simulink model "Optimization_Implementation_Sept1_2021"  (R2021a)
settings: Solver=FixedStepAuto  StartTime=0.0  StopTime=inf  FixedStep=.001  RelTol=1e-3
libraries: speedgoatlib_IO691 x5, canmsglib x4, slrealtimeutilitieslib x2
settings Model: SimulationMode=external  NumberOfSteps=2  Creator=celwe  LastModifiedBy=celwe
settings SolverCC: ConcurrentTasks=on  PositivePriorityOrder=on
settings OptimizationCC: BlockReduction=off  OptimizeBlockIOStorage=off
settings DebuggingCC: TasksWithSamePriorityMsg=none
settings HardwareCC: ProdBitPerLong=64  ProdLongLongMode=on  ProdHWDeviceType=Intel->x86-64 (Linux 64)
settings RTWCC: Description=Simulink Real-Time  SystemTargetFile=slrealtime.tlc  TemplateMakefile=slrealtime_default_tmf  Toolchain=Simulink Real-Time Toolchain  BuildConfiguration=Faster Runs  CodeExecutionProfiling=on  TargetLang=C++

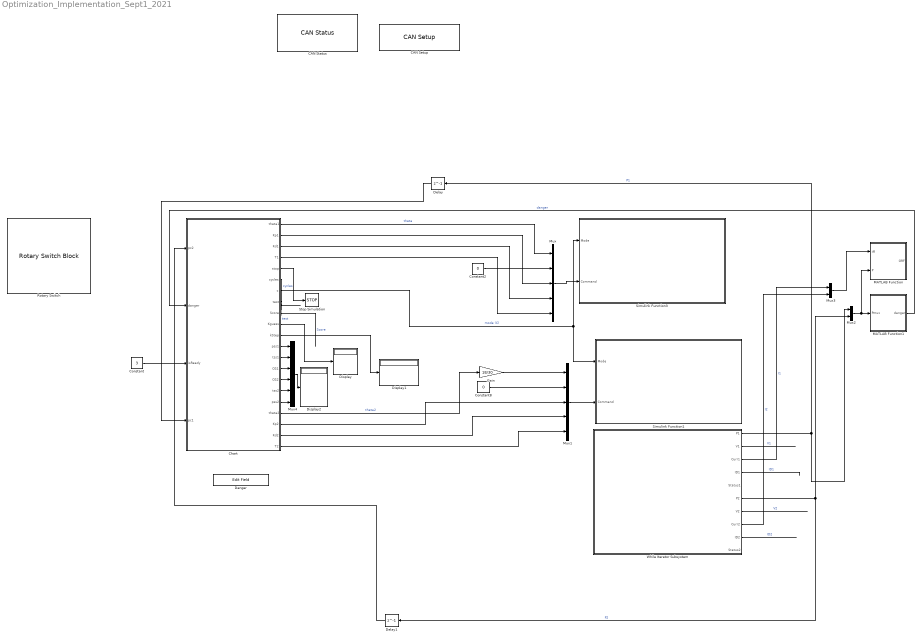
== system Optimization_Implementation_Sept1_2021 ==
  "CAN Setup " : speedgoatlib_IO691/CAN Setup   moduletype=IO691  id=1  pciSlot=-1  chn1=CAN (HS)  chn2=CAN (HS)  chn3=Disabled  chn4=Disabled  initStruct=[]  termStruct=[]  ArbitrationbdrChn1=1.0 MBaud  ArbitrationManbdrChn1=[2,8,31,8]  FdbdrChn1=5.0 MBaud  FdManbdrChn1=[2,2,5,2]  ArbitrationbdrChn2=1.0 MBaud  ArbitrationManbdrChn2=[2,8,31,8]  FdbdrChn2=5.0 MBaud  FdManbdrChn2=[2,2,5,2]  ArbitrationbdrChn3=1.0 MBaud  ArbitrationManbdrChn3=[2,8,31,8]  FdbdrChn3=5.0 MBaud  FdManbdrChn3=[2,2,5,2]  ArbitrationbdrChn4=1.0 MBaud  ArbitrationManbdrChn4=[2,8,31,8]  FdbdrChn4=5.0 MBaud  FdManbdrChn4=[2,2,5,2]  moduleInitValues=[691 1 -1 -1]
      settings: SourceProductName=Simulink Real-Time: Speedgoat I/O Blockset
  CAN Status : speedgoatlib_IO691/CAN Status  moduleId=1  sampleTime=-1  channel=1  busRecovery=Off  arrayOutput=off  controllerCpuLoad=off  controllerLiveCount=off  initModeAct=off  avgBusLoad=off  receiving=off  RxQueueEmpty=off  dataOverrunRcv=off  rxBufferLevel=off  txPending=off  dataOverrunTx=off  txBufferLevel=off  errWarnLimit=off  errPassLimit=off  errBusOff=off  busRecoveryCounter=off  busCouplingErr=off  transceiverErr=off  opMode=off  brp=off  timeSegment1=off  timeSegment2=off  synchronisationJumpWidth=off  dataTSEG1=off  dataTSEG2=off  dataSJW=off  moduleType=691  qtyStatBlk=1  ptIdx=0  isFDMod=0
      settings: SourceProductName=Simulink Real-Time: Speedgoat I/O Blockset
  Chart : Stateflow chart  TreatAsAtomicUnit=on
      settings: PortSchema="{\"entries\":[{\"content\":{\"sides\":[{\"content\":{\"connectorIds\":[\"In1\",\"In2\",\"In3\",\"In4\"]},\"type\":\"ConnectorPlacement.EquallySpacedRectSide\",\"uuid\":\"09499f21-f50c-4ce4-914e-8b9942bcc246\"},{\"content\":{\"connectorIds\":[\"Out2\",\"Out7\",\"Out9\",\"Out5\",\"Out1\",\"Out11\",\"Out4\",\"Out12\",\"Out13\",\"Out14\",\"Out15\",\"Out16\",\"Out17\",\"Out18\",\"Out19\",\"Out20\",\"Out21\",\"Out3\",\"Out8\",\"Out10\",\"Out6\"],\"side\":\"RIGHT\"},\"type\":\"ConnectorPlacement.EquallySpacedRectSide\",\"uuid\":\"b935e908-ace3-4dfb-ad6d-08dfed6ffdb3\"},{\"content\":{\"connectorIds\":[],\"side\":\"TOP\"},\"type\":\"ConnectorPlacement.EquallySpacedRectSide\",\"uuid\":\"4cd7c5d6-1f1f-4a1f-84b4-9b198395645e\"}]},\"type\":\"ConnectorPlacement.EquallySpacedConnector\",\"uuid\":\"2dc6a8af-05a8-4f21-87ab-6863f156f450\"}],\"packageUris\":[\"http://schema.mathworks.com/mf0/Connector/R2020b\"],\"version\":\"1.0\"}"
  Constant : Constant  Value=3
  Constant2 : Constant  Value=0
  Constant8 : Constant  Value=0
  Danger : EditField  LabelPosition=Hide  ShowInitialText=on  Alignment=Center
  Delay : Delay  DelayLength=1
  Delay1 : Delay  DelayLength=1
  Display : Display
  Display1 : Display
  Display2 : Display
  Gain : Gain  Gain=18/30
  MATLAB Function : MATLAB Function  TreatAsAtomicUnit=on
  MATLAB Function1 : MATLAB Function  TreatAsAtomicUnit=on
  Mux : Mux  Inputs=5
  Mux1 : Mux  Inputs=5
  Mux2 : Mux  Inputs=2
  Mux3 : Mux  Inputs=2
  Mux4 : Mux  Inputs=6
  Rotary Switch : RotarySwitchBlock
      settings: Values={{'Zeroing', 'Initiated', 'Stand', 'Jumping', 'deInit', 'Idle'}, [0 1 2 3 4 5]}
  Simulink Function1 : Subsystem  TreatAsAtomicUnit=on
  Simulink Function3 : Subsystem  TreatAsAtomicUnit=on
  Stop Simulation : Stop
  While Iterator Subsystem : Subsystem  TreatAsAtomicUnit=on
  wires:
  Mux/1 -> Simulink Function3/2(Command)
  Constant2/1 -> Mux/2
  Chart/7(Kp1) -> Mux/3
  Chart/9(Kd1) -> Mux/4
  Chart/5(T1) -> Mux/5
  Chart/10(Kd2) -> Mux1/4
  Constant8/1 -> Mux1/2
  Mux1/1 -> Simulink Function1/2(Command)
  Chart/8(Kp2) -> Mux1/3
  Chart/4(c) -> Simulink Function1/1(Mode), Simulink Function3/1(Mode)  "mode (C)"
  Chart/6(T2) -> Mux1/5
  Mux2/1 -> MATLAB Function/2(P), MATLAB Function1/1(Pmux)
  MATLAB Function1/1(danger) -> Chart/2(danger)  "danger"
  Chart/2(theta1) -> Mux/1  "theta"
  Gain/1 -> Mux1/1
  Chart/3(theta2) -> Gain/1  "theta2"
  While Iterator Subsystem/1(P1) -> Mux2/1, Delay/1  "P1"
  While Iterator Subsystem/2(V1) -> ?  "V1"
  While Iterator Subsystem/3(Curr1) -> Mux3/1  "I1"
  While Iterator Subsystem/4(ID1) -> ?  "ID1"
  While Iterator Subsystem/6(P2) -> Delay1/1, Mux2/2  "P2"
  While Iterator Subsystem/7(V2) -> ?  "V2"
  While Iterator Subsystem/8(Curr2) -> Mux3/2  "I2"
  While Iterator Subsystem/9(ID2) -> ?  "ID2"
  Mux3/1 -> MATLAB Function/1(Iff)
  Chart/1(stop) -> Stop Simulation/1
  Delay1/1 -> Chart/1(pc2)
  Constant/1 -> Chart/3(isReady)
  Delay/1 -> Chart/4(pc1)
  Chart/11(cycles) -> ?  "cycles"
  Chart/12(test) -> ?  "test"
  Chart/13(Score) -> ?  "Score"
  Chart/14(Kguess) -> Display/1
  Chart/15(kStep) -> Display1/1
  Chart/16(pss1) -> Mux4/1
  Chart/17(tss1) -> Mux4/2
  Chart/18(OS1) -> Mux4/3
  Chart/19(OS2) -> Mux4/4
  Chart/20(tss2) -> Mux4/5
  Chart/21(pss2) -> Mux4/6
  Mux4/1 -> Display2/1

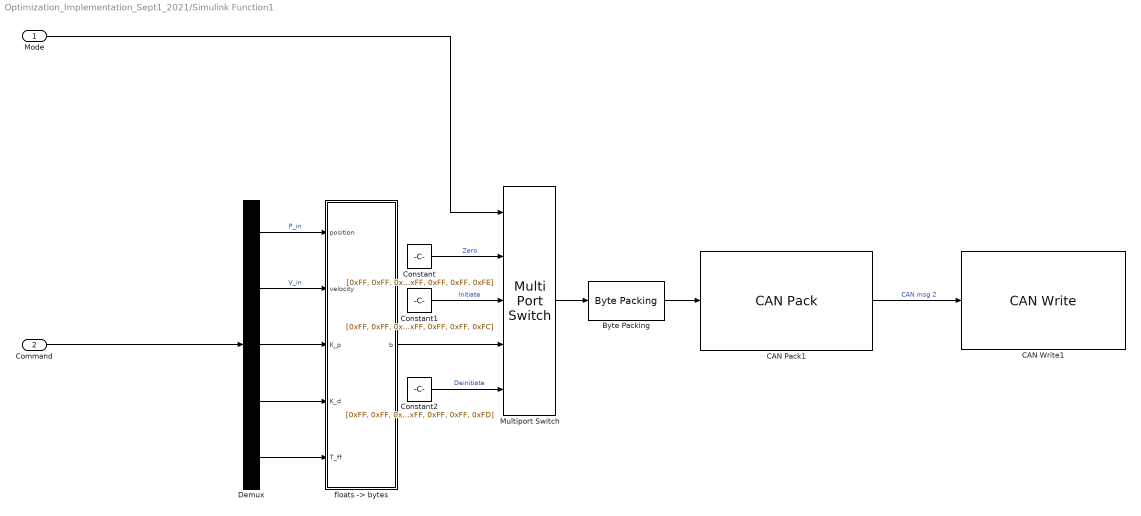
== system Optimization_Implementation_Sept1_2021/Simulink Function1 ==
  Mode : Inport
  Command : Inport  Port=2
  Byte Packing : slrealtimeutilitieslib/Byte Packing  MaskPackedDataType=uint8  MaskUnpackedDataTypes={['uint8']}  MaskAlignment=1
  CAN Pack1 : canmsglib/CAN Pack  MsgList=(none)  MsgName=CAN Msg  MsgIDType=Standard (11-bit identifier)  MsgIdentifier=2  MsgLength=8  Remote=off  ApplyMinMax=off  BusOutput=off  SignalInfo={ 'b1', '0', '8', 'LE', 'unsigned', 'Standard', '0', '1', '0', '-Inf', 'Inf'; 'b2', '8', '8', 'LE', 'unsigned', 'Standard', '0', '1', '0', '-Inf', 'Inf'; 'b3', '16', '8', 'LE', 'unsigned', 'Standard', '0', '1', '0', '-Inf', 'Inf'; 'b4', '24', '8', 'LE', 'unsigned', 'Standard', '0', '1', '0', '-Inf', 'Inf'; 'b5', '32', '8', 'LE', 'unsigned', 'Standard', '0', '1', '0', '-Inf', 'Inf'; 'b6', '40', '8', 'LE', 'unsigned', 'Standard', '0', '1', '0', '-Inf', 'Inf'; 'b7', '48', '8', 'LE', 'unsigned', 'Standard', '0', '1', '0', '-Inf', 'Inf'; 'b8', '56', '8', 'LE', 'unsigned', 'Standard', '0', '1', '0', '-Inf', 'Inf' }
      settings: SourceProductBaseCode=ME,XP,VN  DataFormat=raw data
  CAN Write1 : speedgoatlib_IO691/CAN Write  id=1  ts=-1  channel=1  messageType=CAN  enableStatusPort=off  canType=CAN (HS)  initValues=[691 1 -1 0 1 1 0]
      settings: SourceProductName=Simulink Real-Time: Speedgoat I/O Blockset
  Constant : Constant  Value=[0xFF, 0xFF, 0xFF, 0xFF, 0xFF, 0xFF, 0xFF, 0xFE]
  Constant1 : Constant  Value=[0xFF, 0xFF, 0xFF, 0xFF, 0xFF, 0xFF, 0xFF, 0xFC]
  Constant2 : Constant  Value=[0xFF, 0xFF, 0xFF, 0xFF, 0xFF, 0xFF, 0xFF, 0xFD]
  Demux : Demux  Outputs=5
  Multiport Switch : MultiPortSwitch  Inputs=4  DiagnosticForDefault=None
  "floats -> bytes" : MATLAB Function  TreatAsAtomicUnit=on
  wires:
  Demux/5 -> "floats -> bytes"/5(T_ff)
  Multiport Switch/1 -> Byte Packing/1
  Demux/4 -> "floats -> bytes"/4(K_d)
  Demux/1 -> "floats -> bytes"/1(position)  "P_in"
  Constant/1 -> Multiport Switch/2  "Zero"
  Demux/2 -> "floats -> bytes"/2(velocity)  "V_in"
  Constant2/1 -> Multiport Switch/5  "Deinitiate"
  CAN Pack1/1 -> CAN Write1/1  "CAN msg 2"
  Byte Packing/1 -> CAN Pack1/1
  Constant1/1 -> Multiport Switch/3  "Initiate"
  "floats -> bytes"/1(b) -> Multiport Switch/4
  Demux/3 -> "floats -> bytes"/3(K_p)
  Mode/1 -> Multiport Switch/1
  Command/1 -> Demux/1

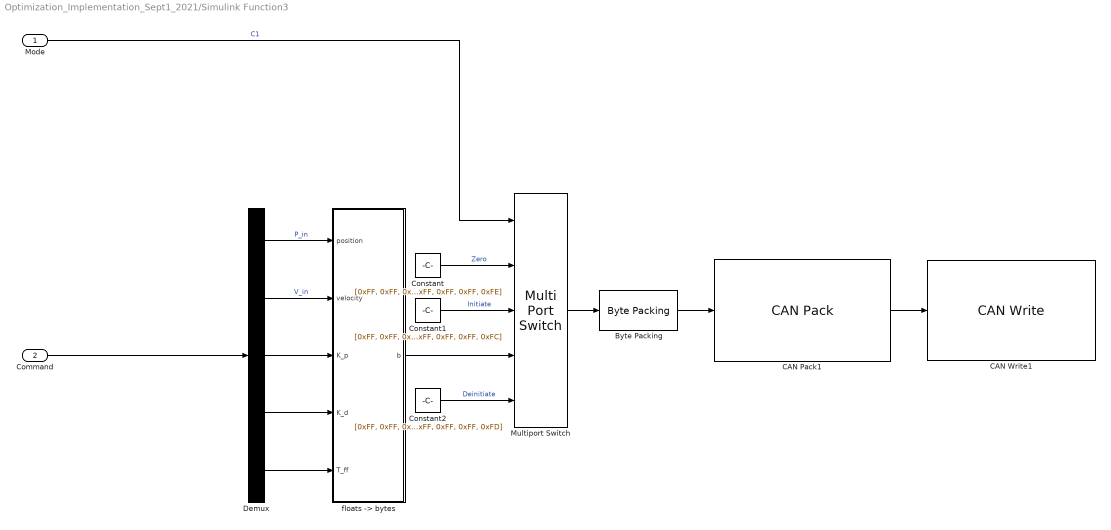
== system Optimization_Implementation_Sept1_2021/Simulink Function3 ==
  Mode : Inport
  Command : Inport  Port=2
  Byte Packing : slrealtimeutilitieslib/Byte Packing  MaskPackedDataType=uint8  MaskUnpackedDataTypes={['uint8']}  MaskAlignment=1
  CAN Pack1 : canmsglib/CAN Pack  MsgList=(none)  MsgName=CAN Msg  MsgIDType=Standard (11-bit identifier)  MsgIdentifier=1  MsgLength=8  Remote=off  ApplyMinMax=off  BusOutput=off  SignalInfo={ 'b1', '0', '8', 'LE', 'unsigned', 'Standard', '0', '1', '0', '-Inf', 'Inf'; 'b2', '8', '8', 'LE', 'unsigned', 'Standard', '0', '1', '0', '-Inf', 'Inf'; 'b3', '16', '8', 'LE', 'unsigned', 'Standard', '0', '1', '0', '-Inf', 'Inf'; 'b4', '24', '8', 'LE', 'unsigned', 'Standard', '0', '1', '0', '-Inf', 'Inf'; 'b5', '32', '8', 'LE', 'unsigned', 'Standard', '0', '1', '0', '-Inf', 'Inf'; 'b6', '40', '8', 'LE', 'unsigned', 'Standard', '0', '1', '0', '-Inf', 'Inf'; 'b7', '48', '8', 'LE', 'unsigned', 'Standard', '0', '1', '0', '-Inf', 'Inf'; 'b8', '56', '8', 'LE', 'unsigned', 'Standard', '0', '1', '0', '-Inf', 'Inf' }
      settings: SourceProductBaseCode=ME,XP,VN  DataFormat=raw data
  CAN Write1 : speedgoatlib_IO691/CAN Write  id=1  ts=-1  channel=1  messageType=CAN  enableStatusPort=off  canType=CAN (HS)  initValues=[691 1 -1 0 1 1 0]
      settings: SourceProductName=Simulink Real-Time: Speedgoat I/O Blockset
  Constant : Constant  Value=[0xFF, 0xFF, 0xFF, 0xFF, 0xFF, 0xFF, 0xFF, 0xFE]
  Constant1 : Constant  Value=[0xFF, 0xFF, 0xFF, 0xFF, 0xFF, 0xFF, 0xFF, 0xFC]
  Constant2 : Constant  Value=[0xFF, 0xFF, 0xFF, 0xFF, 0xFF, 0xFF, 0xFF, 0xFD]
  Demux : Demux  Outputs=5
  Multiport Switch : MultiPortSwitch  Inputs=4  DiagnosticForDefault=None
  "floats -> bytes" : MATLAB Function  TreatAsAtomicUnit=on
  wires:
  Demux/5 -> "floats -> bytes"/5(T_ff)
  Multiport Switch/1 -> Byte Packing/1
  Demux/4 -> "floats -> bytes"/4(K_d)
  Demux/1 -> "floats -> bytes"/1(position)  "P_in"
  Constant/1 -> Multiport Switch/2  "Zero"
  Demux/2 -> "floats -> bytes"/2(velocity)  "V_in"
  Constant2/1 -> Multiport Switch/5  "Deinitiate"
  CAN Pack1/1 -> CAN Write1/1
  Byte Packing/1 -> CAN Pack1/1
  Constant1/1 -> Multiport Switch/3  "Initiate"
  "floats -> bytes"/1(b) -> Multiport Switch/4
  Demux/3 -> "floats -> bytes"/3(K_p)
  Mode/1 -> Multiport Switch/1  "C1"
  Command/1 -> Demux/1

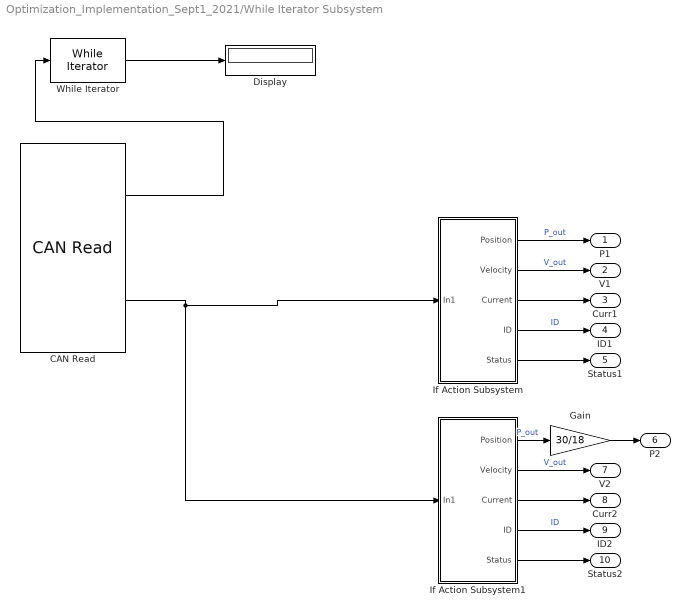
== system Optimization_Implementation_Sept1_2021/While Iterator Subsystem ==
  CAN Read : speedgoatlib_IO691/CAN Read  id=1  ts=-1  channel=1  messageType=CAN  canType=CAN (HS)  initValues=[691 1 -1 0 1 1]
      settings: SourceProductName=Simulink Real-Time: Speedgoat I/O Blockset
  Display : Display
  Gain : Gain  Gain=30/18
  If Action Subsystem : Subsystem  TreatAsAtomicUnit=on
  If Action Subsystem1 : Subsystem  TreatAsAtomicUnit=on
  While Iterator : WhileIterator  MaxIters=-1  WhileBlockType=do-while  ResetStates=reset  ShowIterationPort=on
  P1 : Outport
  V1 : Outport  Port=2
  Curr1 : Outport  Port=3
  ID1 : Outport  Port=4
  Status1 : Outport  Port=5
  P2 : Outport  Port=6
  V2 : Outport  Port=7
  Curr2 : Outport  Port=8
  ID2 : Outport  Port=9
  Status2 : Outport  Port=10
  wires:
  CAN Read/1 -> While Iterator/1
  CAN Read/2 -> If Action Subsystem1/1(In1), If Action Subsystem/1(In1)
  If Action Subsystem/1(Position) -> P1/1  "P_out"
  If Action Subsystem/2(Velocity) -> V1/1  "V_out"
  If Action Subsystem/3(Current) -> Curr1/1
  If Action Subsystem/4(ID) -> ID1/1  "ID"
  If Action Subsystem/5(Status) -> Status1/1
  If Action Subsystem1/5(Status) -> Status2/1
  If Action Subsystem1/4(ID) -> ID2/1  "ID"
  If Action Subsystem1/3(Current) -> Curr2/1
  If Action Subsystem1/2(Velocity) -> V2/1  "V_out"
  While Iterator/1 -> Display/1
  Gain/1 -> P2/1
  If Action Subsystem1/1(Position) -> Gain/1  "P_out"

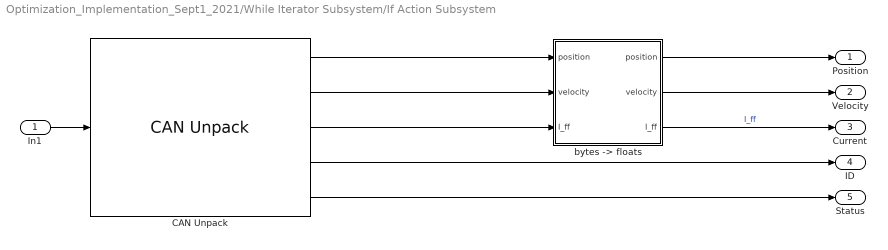
== system Optimization_Implementation_Sept1_2021/While Iterator Subsystem/If Action Subsystem ==
  In1 : Inport
  CAN Unpack : canmsglib/CAN Unpack  MsgList=(none)  MsgName=CAN Msg  MsgIDType=Standard (11-bit identifier)  MsgIdentifier=1  MsgLength=6  SignalInfo={ 'position', '16', '16', 'BE', 'unsigned', 'Standard', '0', '1', '0', '0', '65535'; 'velocity', '36', '12', 'BE', 'unsigned', 'Standard', '0', '1', '0', '0', '4095'; 'current', '40', '12', 'BE', 'unsigned', 'Standard', '0', '1', '0', '0', '4095'; 'id', '0', '8', 'BE', 'unsigned', 'Standard', '0', '1', '0', '0', '255' }  IDPort=off  TimestampPort=off  ErrorPort=off  RemotePort=off  LengthPort=off  StatusPort=on  ApplyMinMax=off
      settings: SourceProductBaseCode=ME,XP,VN
  "bytes -> floats" : MATLAB Function  TreatAsAtomicUnit=on
  Position : Outport
  Velocity : Outport  Port=2
  Current : Outport  Port=3
  ID : Outport  Port=4
  Status : Outport  Port=5
  wires:
  CAN Unpack/5 -> Status/1
  CAN Unpack/3 -> "bytes -> floats"/3("I_ff ")
  CAN Unpack/4 -> ID/1
  "bytes -> floats"/2(velocity) -> Velocity/1
  "bytes -> floats"/3(I_ff) -> Current/1  "I_ff"
  CAN Unpack/2 -> "bytes -> floats"/2("velocity ")
  In1/1 -> CAN Unpack/1
  CAN Unpack/1 -> "bytes -> floats"/1("position ")
  "bytes -> floats"/1(position) -> Position/1

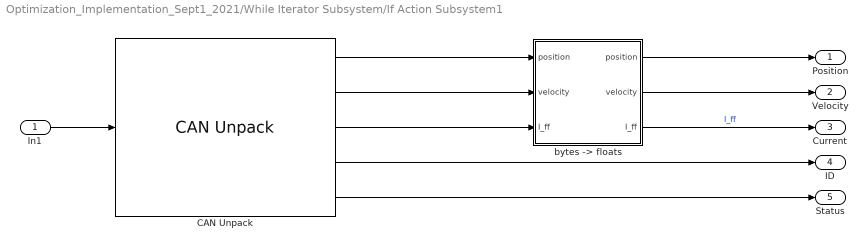
== system Optimization_Implementation_Sept1_2021/While Iterator Subsystem/If Action Subsystem1 ==
  In1 : Inport
  CAN Unpack : canmsglib/CAN Unpack  MsgList=(none)  MsgName=CAN Msg  MsgIDType=Standard (11-bit identifier)  MsgIdentifier=2  MsgLength=6  SignalInfo={ 'position', '16', '16', 'BE', 'unsigned', 'Standard', '0', '1', '0', '0', '65535'; 'velocity', '36', '12', 'BE', 'unsigned', 'Standard', '0', '1', '0', '0', '4095'; 'current', '40', '12', 'BE', 'unsigned', 'Standard', '0', '1', '0', '0', '4095'; 'id', '0', '8', 'BE', 'unsigned', 'Standard', '0', '1', '0', '0', '255' }  IDPort=off  TimestampPort=off  ErrorPort=off  RemotePort=off  LengthPort=off  StatusPort=on  ApplyMinMax=off
      settings: SourceProductBaseCode=ME,XP,VN
  "bytes -> floats" : MATLAB Function  TreatAsAtomicUnit=on
  Position : Outport
  Velocity : Outport  Port=2
  Current : Outport  Port=3
  ID : Outport  Port=4
  Status : Outport  Port=5
  wires:
  CAN Unpack/5 -> Status/1
  CAN Unpack/1 -> "bytes -> floats"/1("position ")
  CAN Unpack/3 -> "bytes -> floats"/3("I_ff ")
  "bytes -> floats"/1(position) -> Position/1
  CAN Unpack/4 -> ID/1
  "bytes -> floats"/2(velocity) -> Velocity/1
  "bytes -> floats"/3(I_ff) -> Current/1  "I_ff"
  CAN Unpack/2 -> "bytes -> floats"/2("velocity ")
  In1/1 -> CAN Unpack/1

== matlab function Optimization_Implementation_Sept1_2021/While Iterator Subsystem/If Action Subsystem1/bytes -> floats ==
  data: position input; position output; velocity output; I_ff output; velocity input; I_ff input
function [position, velocity, I_ff] = fcn(position, velocity, I_ff)

P_MIN  =-95.5;  % [rad]
P_MAX  = 95.5;  % [rad]
V_MIN  =-45;    % [rad/s]
V_MAX  = 45;    % [rad/s]
I_MIN  =-40;    % []
I_MAX  = 40;    % []

position = position*(P_MAX  - P_MIN)/65535+ P_MIN;
velocity = velocity*(V_MAX  - V_MIN)/4095 + V_MIN;
I_ff     = I_ff*(I_MAX  - I_MIN)/4095 + I_MIN;

== matlab function Optimization_Implementation_Sept1_2021/While Iterator Subsystem/If Action Subsystem/bytes -> floats ==
  data: position input; position output; velocity output; I_ff output; velocity input; I_ff input
function [position, velocity, I_ff] = fcn(position, velocity, I_ff)

P_MIN  =-95.5;  % [rad]
P_MAX  = 95.5;  % [rad]
V_MIN  =-45;    % [rad/s]
V_MAX  = 45;    % [rad/s]
I_MIN  =-40;    % []
I_MAX  = 40;    % []

position = position*(P_MAX  - P_MIN)/65535+ P_MIN;
velocity = velocity*(V_MAX  - V_MIN)/4095 + V_MIN;
I_ff     = I_ff*(I_MAX  - I_MIN)/4095 + I_MIN;

== matlab function Optimization_Implementation_Sept1_2021/Simulink Function1/floats -> bytes ==
  data: position input; b output uint8 size=8; velocity input; K_p input; K_d input; T_ff input
function b = fcn(position, velocity, K_p, K_d, T_ff)

P_MIN  =-95.5;  % [rad]
P_MAX  = 95.5;  % [rad]
V_MIN  =-45;    % [rad/s] 30 to 45
V_MAX  = 45;    % [rad/s]
KP_MIN = 0;     % [Nm/rad]
KP_MAX = 500;   % [Nm/rad]
KD_MIN = 0;     % [Nm*s/rad
KD_MAX = 5;     % [Nm*s/rad
T_MIN  =-18;    % [Nm]
T_MAX  = 18;    % [Nm]

position = floor((max(min(position,P_MAX) ,P_MIN)  - P_MIN )*65535/(P_MAX  - P_MIN));
velocity = floor((max(min(velocity,V_MAX) ,V_MIN)  - V_MIN )*4095 /(V_MAX  - V_MIN));
K_p      = floor((max(min(K_p     ,KP_MAX),KP_MIN) - KP_MIN)*4095 /(KP_MAX - KP_MIN));
K_d      = floor((max(min(K_d     ,V_MAX) ,V_MIN)  - KD_MIN)*4095 /(KD_MAX - KD_MIN));
T_ff     = floor((max(min(T_ff    ,V_MAX) ,V_MIN)  - T_MIN )*4095 /(T_MAX  - T_MIN));

p  = dec2bin(position);
p  = [repmat('0', 1, 16-length(p)),p];
v  = dec2bin(velocity);
v  = [repmat('0', 1, 12-length(v)),v];
kp = dec2bin(K_p);
kp  = [repmat('0', 1, 12-length(kp)),kp];
kd = dec2bin(K_d);
kd  = [repmat('0', 1, 12-length(kd)),kd];
t  = dec2bin(T_ff);
t  = [repmat('0', 1, 12-length(t)),t];

B = repmat('0', 8, 8);

B(1,:) = p(1:8);
B(2,:) = p(9:16);
B(3,:) = v(1:8);
B(4,:) = [v(9:12),kp(1:4)];
B(5,:) = kp(5:12);
B(6,:) = kd(1:8);
B(7,:) = [kd(9:12),t(1:4)];
B(8,:) = t(5:12);

B  = bin2dec(B);

b = uint8(B);

== matlab function Optimization_Implementation_Sept1_2021/MATLAB Function ==
  data: Iff input; P input; GRF output
function GRF = isGRF(Iff,P)
    GRF = 0;
    threshhold = 2;
    
    P1 = P(1);
    P2 = P(2);
    
    Iff1 = Iff(1);
    Iff2 = Iff(2);
    
    if(((P1<0 && threshhold<Iff1)&& (P2>0 && -threshhold>Iff2))|| ((P1>0 && -threshhold>Iff1) && (P2<0 && threshhold<Iff2)))
        GRF = 1;
    end

== matlab function Optimization_Implementation_Sept1_2021/Simulink Function3/floats -> bytes ==
  data: position input; b output uint8 size=8; velocity input; K_p input; K_d input; T_ff input
function b = fcn(position, velocity, K_p, K_d, T_ff)

P_MIN  =-95.5;  % [rad]
P_MAX  = 95.5;  % [rad]
V_MIN  =-45;    % [rad/s] 30 to 45
V_MAX  = 45;    % [rad/s]
KP_MIN = 0;     % [Nm/rad]
KP_MAX = 500;   % [Nm/rad]
KD_MIN = 0;     % [Nm*s/rad
KD_MAX = 5;     % [Nm*s/rad
T_MIN  =-18;    % [Nm]
T_MAX  = 18;    % [Nm]

position = floor((max(min(position,P_MAX) ,P_MIN)  - P_MIN )*65535/(P_MAX  - P_MIN));
velocity = floor((max(min(velocity,V_MAX) ,V_MIN)  - V_MIN )*4095 /(V_MAX  - V_MIN));
K_p      = floor((max(min(K_p     ,KP_MAX),KP_MIN) - KP_MIN)*4095 /(KP_MAX - KP_MIN));
K_d      = floor((max(min(K_d     ,V_MAX) ,V_MIN)  - KD_MIN)*4095 /(KD_MAX - KD_MIN));
T_ff     = floor((max(min(T_ff    ,V_MAX) ,V_MIN)  - T_MIN )*4095 /(T_MAX  - T_MIN));

p  = dec2bin(position);
p  = [repmat('0', 1, 16-length(p)),p];
v  = dec2bin(velocity);
v  = [repmat('0', 1, 12-length(v)),v];
kp = dec2bin(K_p);
kp  = [repmat('0', 1, 12-length(kp)),kp];
kd = dec2bin(K_d);
kd  = [repmat('0', 1, 12-length(kd)),kd];
t  = dec2bin(T_ff);
t  = [repmat('0', 1, 12-length(t)),t];

B = repmat('0', 8, 8);

B(1,:) = p(1:8);
B(2,:) = p(9:16);
B(3,:) = v(1:8);
B(4,:) = [v(9:12),kp(1:4)];
B(5,:) = kp(5:12);
B(6,:) = kd(1:8);
B(7,:) = [kd(9:12),t(1:4)];
B(8,:) = t(5:12);

B  = bin2dec(B);

b = uint8(B);

== matlab function Optimization_Implementation_Sept1_2021/MATLAB Function1 ==
  data: Pmux input; danger output
function danger = isDanger(Pmux)
    % Pmux position matrix radians
    %       [p(ID1),p(ID2),p(ID3),p(IDN)]

    
    p1Max = 2; 
    p1Min = -2;
    p2Max = 2;
    p2Min = -2;
    
    P1 = Pmux(1:2:end);
    P2 = Pmux(2:2:end);
       
    danger = 0;
    if((0<sum([P1>p1Max] + [P1<p1Min] - [P1<=-95.5])) || (0<sum([P2>p2Max] + [P2<p2Min] - [P2<=-95.5])))
        danger = 1;
    end

== stateflow chart Optimization_Implementation_Sept1_2021/Chart ==
  state Start
  state Zero
    entry:
    c = 1;
  state Init
    entry:
    c = 2;
  state Command
    entry:
    c = 3;
    test = 1;
    cycles = 0;
    Kguess = [22.75,17.10,.92,1.41];
    Ksaved = [0,0,0,0];
    kStep = [-.4,-.4,-.08,.08];
    oldScore = [0,0,0,0];
    oldScoreSlope = [0,0,0,0];
    a1 = 0; b1 = 0; c1 = 0; d1 = 0; e1 = 0;
    state Stand
      entry:
      Kp1= 10;
      Kp2 = 10;
      Kd1= 1;
      Kd2 = 1;
      to = t;
      tstep = 3;
      theta1 = pc1;
      po1 = theta1;
      slope1 = (theta1Release - po1)/tstep;
      theta2 = pc2;
      po2 = theta2;
      slope2 = (theta2Release - po2)/tstep;
      during:
      theta1 = po1 + slope1*(t-to);
      theta2 = po2 + slope2*(t-to);
    state interpretData
      entry:
      pss1 = pc1-theta1Goal;
      pss2 = pc2-theta2Goal;
      Score = (pss1*10)^2 + (pss2*10)^2 + (10*tss1)^2 + (10*tss2)^2 + (10*OS1^2) + (10*OS2^2) + delt1^2 + delt2^2;
      temp = kStep(test);
      [a1,b1,c1,d1,e1] = Changes(Kguess(test), Ksaved(test), kStep(test), Score,oldScore(test), oldScoreSlope(test));
      Kguess(test) = a1; Ksaved(test) = b1; kStep(test) = c1; oldScore(test) = d1; oldScoreSlope(test) = e1;
      [test, cycles] = testSwitch(test,temp,kStep(test), cycles);
    state Flight
      entry:
      tr = t
      delt1 = 0;
      delt2 = 0;
      OS1 = -pc1;
      OS2 = -pc2;
      tss1 = 0;
      tss2 = 0;
      theta1 = theta1Goal;
      Kp1 = Kguess(1);
      Kd1 = Kguess(3);
      theta2 = theta2Goal;
      Kp2 = Kguess(2);
      Kd2 = Kguess(4);
      during:
      [OS1 delt1 tss1] = Record(theta1Goal-pc1, OS1, t - tr,delt1,tss1,1);
      [OS2 delt2 tss2] = Record(theta2Goal-pc2, OS2, t - tr,delt2,tss2,-1);
    state Idle
    (default) -> Stand
    interpretData -> Stand : [isReady == 3]
    Flight -> interpretData : after(5,sec)
    Stand -> Idle : [(theta1 >= theta1Release & slope1>0) | (theta1 <= theta1Release & slope1<0)]
        | {theta1 = theta1Release; theta2 = theta2Release;}
    Idle -> Flight : [isReady == 3]{after(5,sec)}
  state FinalShutdown
    entry:
    Kp1 = 0;
    Kp2 = 0;
    theta1 = 0;
    theta2 = 0;
    T1 = 0;
    T2 = 0;
  state Deinitiate
    entry:
    c = 4;
  (default) -> Start : {theta1Release = 0.06;
      | theta2Release = -.19;
      | theta1Goal = -0.35;
      | theta2Goal = 0.63;}
  Start -> Init [order 2] : [isReady == 1]
      | {after(3, sec);}
  Start -> Zero [order 1] : [isReady == 0]
  Zero -> Init : [isReady == 1]
      | {after(3,sec);}
  Init -> FinalShutdown [order 2] : [isReady == 4 | danger == 1]
  Init -> Command [order 1] : [isReady == 2]
      | {after(3,sec);}
  Command -> FinalShutdown : [cycles == 5 | isReady == 4 | danger == 1]
  (junction 36) -> Deinitiate : {stop = 1;}
  Deinitiate -> (junction 36) : after(3,sec)
  FinalShutdown -> Deinitiate
  data: K function_input; KOld function_input; KGuess function_output; Ko function_output; kStepOut function_output; kStepIn function_input; S function_input; oldS function_input; oldSSlope function_input; newS function_output; Sdot function_output; testN function_input; old function_input; new function_input; Ntest function_output; count function_output; countN function_input; delp function_input; OSin function_input; deltin function_input; deltold function_input; OSout function_output; deltout function_output; tss function_input; tssOut function_output; sign function_input; stop output =0; theta1 output; theta2 output; c output; tstep local; to local; pc2 input; T1 output =0; T2 output =0; Kp1 output =25; Kp2 output =25; Kd1 output =.1; Kd2 output =.1; po1 local; po2 local; slope1 local; slope2 local; danger input; isReady input; pc1 input; theta1Release local; theta1Goal local; theta2Goal local; theta2Release local; Ksaved local; a1 local; b1 local; c1 local; d1 local; delt1 local; delt2 local; e1 local; oldScore local; oldScoreSlope local; temp local; tr local; cycles output; test output; Score output; Kguess output; kStep output; pss1 output; tss1 output; OS1 output; OS2 output; tss2 output; pss2 output
  function [KGuess, Ko, kStepOut,newS,Sdot] = Changes(K, KOld, kStepIn, S,oldS, oldSSlope):
    | function [KGuess, Ko, kStepOut,newS,Sdot] = Changes(K, KOld, kStepIn, S,oldS, oldSSlope)
    | 
    | if(oldS == 0)
    |     Ko = K;
    |     kStepOut = kStepIn;
    |     newS = S; 
    |     Sdot = 0;
    |     KGuess = Ko + kStepOut;
    | elseif(oldSSlope == 0)
    |     Sdot = (S - oldS)/kStep(test);
    |     if(S <= oldS)
    |         Ko = K;
    |         kStepOut = kStepIn;
    |         newS = S;        
    |     else
    |         Ko = KOld;
    |         kStepOut = -kStepIn;
    |         newS = oldS;
    |     end
    |     KGuess = Ko + kStepOut;
    | else
    |     Sdot = (S - oldS)/kStep(test);
    |     if(sign(Sdot) ~= sign(oldSSlope))
    |         kStepIn = kStepIn/2;
    |     end
    |     
    |     if(S <= oldS)
    |         Ko = K;
    |         kStepOut = kStepIn;
    |         newS = S;        
    |     else
    |         Ko = KOld;
    |         kStepOut = -kStepIn;
    |         newS = oldS;
    |     end
    |     KGuess = Ko + kStepOut;
    | end
  function [Ntest, count] = testSwitch(testN,old,new,countN):
    | function [Ntest, count] = testSwitch(testN,old,new,countN)
    | count = countN;
    | Ntest = testN;
    | if(abs(old) ~= abs(new))
    |     Ntest = testN + 1;
    |     
    |     if(Ntest == 5)
    |         Ntest = 1;
    |         count = countN + 1;
    |     end
    | end
  function [OSout, deltout,tssOut] = Record(delp,OSin,deltin,deltold,tss,sign):
    | function [OSout, deltout,tssOut] = Record(delp,OSin,deltin,deltold,tss,sign)
    | if delp*sign<OSin*sign
    |     OSout = delp;
    | else
    |     OSout = OSin;
    | end
    | 
    | if OSin*sign <= 0.01
    |     deltout = deltin;
    | else
    |     deltout = deltold;
    | end
    | 
    | if abs(delp) > .01
    |     tssOut = deltin;
    | else
    |     tssOut = tss;
    | end
    | 
    | end
